simulink model "es601_ex02s"  (R2019a)
settings: Solver=FixedStepAuto  StartTime=0.0  StopTime=10  FixedStep=0.001  RelTol=1e-3
values from neighbouring files (symbols this model uses):
  c = 10    [es601_analiseEstado.m]    (also in es601_analiseEstadoHomogeno.m; es601_ex02m.m = 1)
  k = 100    [es601_analiseEstado.m]    (also in es601_analiseEstadoHomogeno.m; es601_ex02m.m = 1000; es601_ex04_02m.m = 0:10; es601_ex05_01m.m = 0:9)
  m = 1    [es601_analiseEstado.m]    (also in es601_analiseEstadoHomogeno.m; es601_ex02m.m)
settings Model: Creator=Admin-PC  LastModifiedBy=Admin-PC

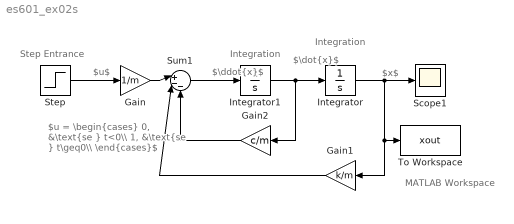
== system es601_ex02s ==
  note: $x$
  note: Step Entrance
  note: Integration
  note: $u = \begin{cases} 0, &\text{se } t<0\\ 1, &\text{se } t\geq0\\ \end{cases}$
  note: $u$
  note: $\dot{x}$
  note: $\ddot{x}$
  note: Integration
  note: MATLAB Workspace
  Gain : Gain  Gain=1/m
  Gain1 : Gain  Gain=k/m
  Gain2 : Gain  Gain=c/m
  Integrator : Integrator
  Integrator1 : Integrator
  Scope1 : Scope
  Step : Step  Time=0  SampleTime=0
  Sum1 : Sum  Inputs=|+--
  To Workspace : ToWorkspace  VariableName=xout  SampleTime=-1
  wires:
  Step/1 -> Gain/1
  Integrator/1 -> Scope1/1, Gain1/1, To Workspace/1
  Gain1/1 -> Sum1/2
  Gain/1 -> Sum1/1
  Sum1/1 -> Integrator1/1
  Integrator1/1 -> Integrator/1, Gain2/1
  Gain2/1 -> Sum1/3
